simulink model "Vehicle_Resistance_Forces_Model_test"  (R2020a)
settings: Solver=VariableStepDiscrete  StartTime=0.0  StopTime=1180  RelTol=1e-3
model workspace (MAT data in the model file):
  acceleration = [0; 1.04; 0; -0.83; 0; 0.69; 0.79; 0; -0.81; 0; 0.69; 0.51; 0.46; 0; -0.52; 0; -0.97; 0; 0; 1.04; 0; -0.83; 0; 0.69; 0.79; 0; -0.81; 0; 0.69; 0.51; 0.46; 0; -0.52; 0; -0.97; 0; 0; 1.04; 0; -0.83; 0; 0.69; 0.79; 0; -0.81; 0; 0.69; 0.51; 0.46; 0; -0.52; 0; -0.97; 0; 0; 1.04; 0; -0.83; 0; 0.69; 0.79; 0; -0.81; 0; 0.69; 0.51; 0.46; 0; -0.52; 0; -0.97; 0; 0; 0.69; 0.51; 0.42; 0.4; 0; -0.69; 0; 0.43; 0; 0.24; 0; 0.28; 0; -0.69; -1.04; -1.39; 0]
undefined symbols (not defined in the file): avgvelocity, duration, h, km, m, s, Time
libraries: simulink x4, aerolibconvert2 x1
settings Model: Creator=akash  LastModifiedBy=akash

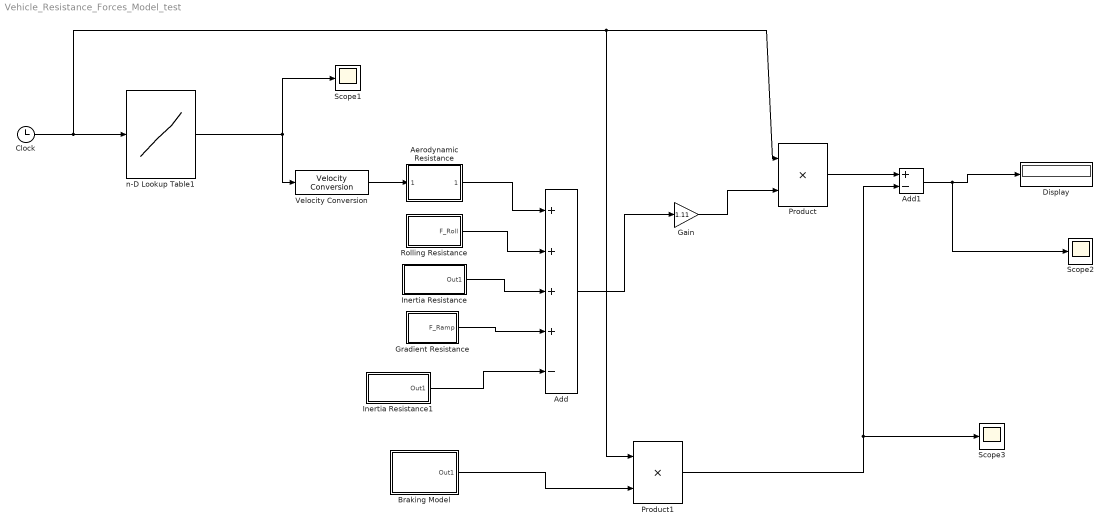
== system Vehicle_Resistance_Forces_Model_test ==
  Add : Sum  Inputs=++++-
  Add1 : Sum  Inputs=+-
  Aerodynamic Resistance : Subsystem
  Braking Model : Subsystem
  Clock : Clock
  Display : Display
  Gain : Gain  Gain=1.11
  Gradient Resistance : Subsystem
  Inertia Resistance : Subsystem
  Inertia Resistance1 : Subsystem
  Product : Product
  Product1 : Product
  Rolling Resistance : Subsystem
  Scope1 : Scope
  Scope2 : Scope
  Scope3 : Scope
  Velocity Conversion : aerolibconvert2/Velocity Conversion  IU=km/h  OU=m/s
  n-D Lookup Table1 : Lookup_n-D  NumberOfTableDimensions=1  BreakpointsForDimension1=Time  BreakpointsForDimension2=acceleration  BreakpointsForDimension3=duration  Table=avgvelocity  InternalRulePriority=Speed  RndMeth=Simplest  InputSameDT=on
  wires:
  n-D Lookup Table1/1 -> Scope1/1, Velocity Conversion/1
  Velocity Conversion/1 -> Aerodynamic Resistance/1(Speed)
  Aerodynamic Resistance/1(F_Aero) -> Add/1
  Rolling Resistance/1(F_Roll) -> Add/2
  Inertia Resistance/1(Out1) -> Add/3
  Gradient Resistance/1(F_Ramp) -> Add/4
  Clock/1 -> n-D Lookup Table1/1, Product1/1, Product/1
  Add/1 -> Gain/1
  Gain/1 -> Product/2
  Inertia Resistance1/1(Out1) -> Add/5
  Braking Model/1(Out1) -> Product1/2
  Product1/1 -> Scope3/1, Add1/2
  Product/1 -> Add1/1
  Add1/1 -> Scope2/1, Display/1

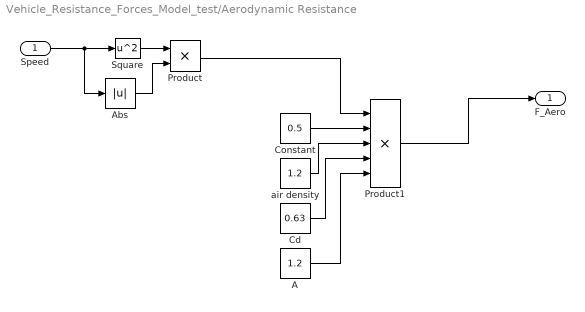
== system Vehicle_Resistance_Forces_Model_test/Aerodynamic Resistance ==
  Speed : Inport
  A : Constant  Value=1.2
  Abs : Abs
  Cd : Constant  Value=0.63
  Constant : Constant  Value=0.5
  Product : Product
  Product1 : Product  Inputs=5
  Square : Math  Operator=square  SaturateOnIntegerOverflow=on
  air density : Constant  Value=1.2
  F_Aero : Outport
  wires:
  air density/1 -> Product1/3
  Product1/1 -> F_Aero/1
  A/1 -> Product1/5
  Speed/1 -> Abs/1, Square/1
  Cd/1 -> Product1/4
  Constant/1 -> Product1/2
  Square/1 -> Product/1
  Abs/1 -> Product/2
  Product/1 -> Product1/1

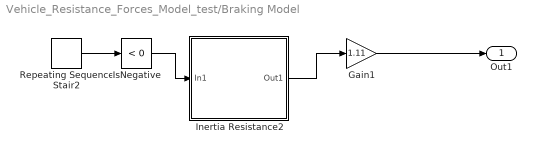
== system Vehicle_Resistance_Forces_Model_test/Braking Model ==
  Gain1 : Gain  Gain=1.11
  Inertia Resistance2 : Subsystem
  IsNegative : simulink/Logic and Bit Operations/Compare To Zero  relop=<  OutDataTypeStr=boolean
  Repeating Sequence Stair2 : simulink/Sources/Repeating Sequence Stair  OutValues=acceleration  tsamp=-1  OutMin=[]  OutMax=[]  OutDataTypeStr=double  OutputDataTypeScalingMode=double  OutDataType=fixdt(0,8)  ConRadixGroup=Best Precision: Vector-wise  OutScaling=2^-12
  Out1 : Outport
  wires:
  Inertia Resistance2/1(Out1) -> Gain1/1
  Repeating Sequence Stair2/1 -> IsNegative/1
  IsNegative/1 -> Inertia Resistance2/1(In1)
  Gain1/1 -> Out1/1

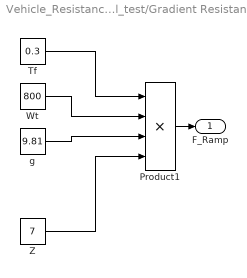
== system Vehicle_Resistance_Forces_Model_test/Gradient Resistance ==
  Product1 : Product  Inputs=4
  Tf : Constant  Value=0.3  VectorParams1D=off  SampleTime=-1
  Wt : Constant  Value=800  VectorParams1D=off  SampleTime=-1
  Z : Constant  Value=7  VectorParams1D=off  SampleTime=-1
  g : Constant  Value=9.81  VectorParams1D=off  SampleTime=-1
  F_Ramp : Outport
  wires:
  g/1 -> Product1/3
  Tf/1 -> Product1/1
  Product1/1 -> F_Ramp/1
  Wt/1 -> Product1/2
  Z/1 -> Product1/4

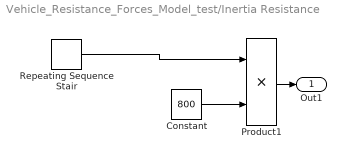
== system Vehicle_Resistance_Forces_Model_test/Inertia Resistance ==
  Constant : Constant  Value=800
  Product1 : Product
  Repeating Sequence Stair : simulink/Sources/Repeating Sequence Stair  OutValues=acceleration  tsamp=-1  OutMin=[]  OutMax=[]  OutDataTypeStr=double  OutputDataTypeScalingMode=double  OutDataType=fixdt(0,8)  ConRadixGroup=Best Precision: Vector-wise  OutScaling=2^-12
  Out1 : Outport
  wires:
  Constant/1 -> Product1/2
  Product1/1 -> Out1/1
  Repeating Sequence Stair/1 -> Product1/1

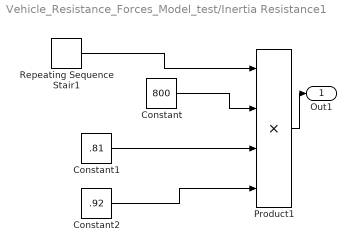
== system Vehicle_Resistance_Forces_Model_test/Inertia Resistance1 ==
  Constant : Constant  Value=800
  Constant1 : Constant  Value=.81
  Constant2 : Constant  Value=.92
  Product1 : Product  Inputs=4
  Repeating Sequence Stair1 : simulink/Sources/Repeating Sequence Stair  OutValues=acceleration  tsamp=-1  OutMin=[]  OutMax=[]  OutDataTypeStr=double  OutputDataTypeScalingMode=double  OutDataType=fixdt(0,8)  ConRadixGroup=Best Precision: Vector-wise  OutScaling=2^-12
  Out1 : Outport
  wires:
  Product1/1 -> Out1/1
  Constant/1 -> Product1/2
  Constant1/1 -> Product1/3
  Constant2/1 -> Product1/4
  Repeating Sequence Stair1/1 -> Product1/1

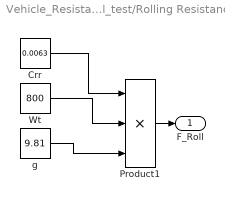
== system Vehicle_Resistance_Forces_Model_test/Rolling Resistance ==
  Crr : Constant  Value=0.0063
  Product1 : Product  Inputs=3
  Wt : Constant  Value=800
  g : Constant  Value=9.81
  F_Roll : Outport
  wires:
  g/1 -> Product1/3
  Crr/1 -> Product1/1
  Wt/1 -> Product1/2
  Product1/1 -> F_Roll/1

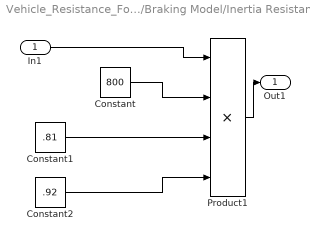
== system Vehicle_Resistance_Forces_Model_test/Braking Model/Inertia Resistance2 ==
  In1 : Inport
  Constant : Constant  Value=800
  Constant1 : Constant  Value=.81
  Constant2 : Constant  Value=.92
  Product1 : Product  Inputs=4
  Out1 : Outport
  wires:
  Constant2/1 -> Product1/4
  Constant1/1 -> Product1/3
  Constant/1 -> Product1/2
  In1/1 -> Product1/1
  Product1/1 -> Out1/1
